simulink model "Lab2_Task_4"  (R2023b)
settings: Solver=FixedStepDiscrete  StartTime=0.0  StopTime=Inf  FixedStep=0.02  RelTol=1e-3  EnableMultiTasking=on
model workspace (MAT data in the model file):
  SL_ROS_VariableLengthArrays_MaxSizes.CommonInfo.ArrayTruncateAction = 'EmitWarning'
  SL_ROS_VariableLengthArrays_MaxSizes.MsgTypeMap = containers.Map
  SL_ROS_VariableLengthArrays_MaxSizes.MsgTypeMap.serialization.keys = {'sensor_msgs/LaserScan'}
  SL_ROS_VariableLengthArrays_MaxSizes.MsgTypeMap.serialization.values{1}(1).PropertyName = 'Intensities'
  SL_ROS_VariableLengthArrays_MaxSizes.MsgTypeMap.serialization.values{1}(1).DataType = 'single'
  SL_ROS_VariableLengthArrays_MaxSizes.MsgTypeMap.serialization.values{1}(1).MaxLength = 360
  SL_ROS_VariableLengthArrays_MaxSizes.MsgTypeMap.serialization.values{1}(2).PropertyName = 'Ranges'
  SL_ROS_VariableLengthArrays_MaxSizes.MsgTypeMap.serialization.values{1}(2).DataType = 'single'
  SL_ROS_VariableLengthArrays_MaxSizes.MsgTypeMap.serialization.values{1}(2).MaxLength = 360
  SL_ROS_VariableLengthArrays_MaxSizes.MsgTypeMap.serialization.uniformity = 0
  SL_ROS_VariableLengthArrays_MaxSizes.MsgTypeMap.serialization.keyType = 'char'
  SL_ROS_VariableLengthArrays_MaxSizes.MsgTypeMap.serialization.valueType = 'any'
undefined symbols (not defined in the file or in its folder): angdiff, Angular, DiscIntNeverNeededParam, Linear
libraries: robotlib x3, simulink_extras x2, robotcorelib x1
settings Model: Creator=The MathWorks, Inc.  LastModifiedBy=hampu
settings SolverCC: AlgebraicLoopSolver=TrustRegion
settings DataIOCC: LimitDataPoints=on  SaveFormat=Array  ReturnWorkspaceOutputs=off
settings OptimizationCC: ZeroExternalMemoryAtStartup=off  ZeroInternalMemoryAtStartup=off  LifeSpan=Inf  MaxStackSize=64
settings DebuggingCC: SolverPrmCheckMsg=warning  UnconnectedInputMsg=warning  UnconnectedOutputMsg=warning  UnconnectedLineMsg=warning  AllowSymbolicDim=off  SFUnexpectedBacktrackingDiag=warning  SFNoUnconditionalDefaultTransitionDiag=warning  SFExecutionAtInitializationDiag=none  ArithmeticOperatorsInVariantConditions=warning
settings HardwareCC: ProdBitPerPointer=32  ProdBitPerSizeT=32  ProdBitPerPtrDiffT=32  ProdLargestAtomicFloat=None  ProdIntDivRoundTo=Undefined  ProdEndianess=Unspecified  ProdWordSize=32  ProdHWDeviceType=Generic->Unspecified (assume 32-bit Generic)  TargetHWDeviceType=Generic->Unspecified (assume 32-bit Generic)  UseEmbeddedCoderFeatures=off
settings ModelReferenceCC: EnableRefExpFcnMdlSchedulingChecks=on  PropagateSignalLabelsOutOfModel=off
settings SFSimCC: SimUseLocalCustomCode=off  CustomCodeUndefinedFunction=UseInterfaceOnly  SimTargetLang=C++
settings RTWCC: Description=Embedded Coder  SystemTargetFile=ert.tlc  HardwareBoard=Robot Operating System (ROS)  TemplateMakefile=ert_default_tmf  RTWUseLocalCustomCode=off  Toolchain=Catkin  TargetLang=C++
settings CodeAppCC: StateflowObjectComments=on
settings ERTTargetCC: MultiwordLength=2048  ERTCustomFileBanners=off  CodeInterfacePackaging=C++ class  SupportContinuousTime=on  SupportNonInlinedSFcns=on  RemoveResetFunc=off  SupportVariableSizeSignals=on  ModelStepFunctionPrototypeControlCompliant=off  RootIOFormat=Structure reference  ConvertIfToSwitch=off  SuppressUnreachableDefaultCases=off
settings ConfigComp: CovMetricSettings=dw  CovSaveCumulativeToWorkspaceVar=on  CovSaveSingleToWorkspaceVar=on  CovExternalEMLEnable=off  CovSFcnEnable=off

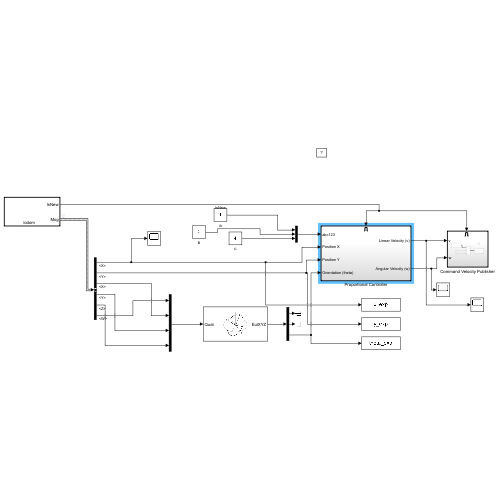
[thumbnail: Simulink's stored preview of the top-level diagram]
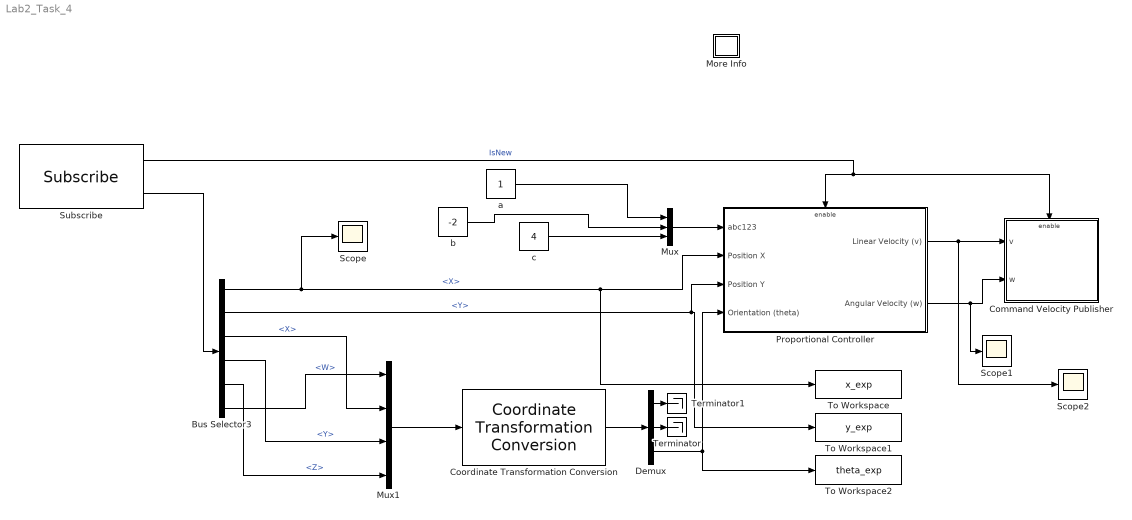
== system Lab2_Task_4 ==
  Bus Selector3 : BusSelector  OutputSignals=Pose.Pose.Position.X,Pose.Pose.Position.Y,Pose.Pose.Orientation.X,Pose.Pose.Orientation.Y,Pose.Pose.Orientation.Z,Pose.Pose.Orientation.W
  Command Velocity Publisher : Subsystem
  Coordinate Transformation Conversion : robotcorelib/Coordinate Transformation Conversion  InputRepresentation=Quaternion  InputEulerSequence=ZYX  ShowTrVecInputPort=on  OutputRepresentation=Euler Angles  OutputEulerSequence=XYZ  ShowTrVecOutputPort=on  SimulateUsing=Interpreted execution
      settings: LibrarySourceBlock=roslib/Utilities/Coordinate Transformation Conversion
  Demux : Demux  Outputs=3
  More Info : Subsystem
      settings: OpenFcn=showdemo(bdroot(gcb))
      mask Display: disp('?')
  Mux : Mux  Inputs=3
  Mux1 : Mux
  Proportional Controller : Subsystem
  Scope : Scope
  Scope1 : Scope
  Scope2 : Scope
  Subscribe : robotlib/Subscribe  topicSource=Select from ROS network  topic=/odom  messageType=nav_msgs/Odometry  SampleTime=-1  legacyBusStruct=off  messageQueueLength=51
  Terminator : Terminator
  Terminator1 : Terminator
  To Workspace : ToWorkspace  VariableName=x_exp  SaveFormat=Timeseries  SampleTime=-1
  To Workspace1 : ToWorkspace  VariableName=y_exp  SaveFormat=Timeseries  SampleTime=-1
  To Workspace2 : ToWorkspace  VariableName=theta_exp  SaveFormat=Timeseries  SampleTime=-1
  a : Constant
  b : Constant  Value=-2
  c : Constant  Value=4
  wires:
  Bus Selector3/5 -> Mux1/4  "<Z>"
  Bus Selector3/1 -> Scope/1, To Workspace/1, Proportional Controller/2(Position X)  "<X>"
  Mux1/1 -> Coordinate Transformation Conversion/1
  Proportional Controller/2(Angular Velocity (w)) -> Scope1/1, Command Velocity Publisher/2(w)
  Bus Selector3/4 -> Mux1/3  "<Y>"
  c/1 -> Mux/3
  Bus Selector3/2 -> To Workspace1/1, Proportional Controller/3(Position Y)  "<Y>"
  Coordinate Transformation Conversion/1 -> Demux/1
  Mux/1 -> Proportional Controller/1(abc123)
  Subscribe/1 -> Command Velocity Publisher/Enable, Proportional Controller/Enable  "IsNew"
  b/1 -> Mux/2
  Demux/2 -> Terminator/1
  Demux/3 -> Proportional Controller/4(Orientation (theta)), To Workspace2/1
  Bus Selector3/6 -> Mux1/1  "<W>"
  Proportional Controller/1(Linear Velocity (v)) -> Scope2/1, Command Velocity Publisher/1(v)
  Demux/1 -> Terminator1/1
  Subscribe/2 -> Bus Selector3/1
  a/1 -> Mux/1
  Bus Selector3/3 -> Mux1/2  "<X>"

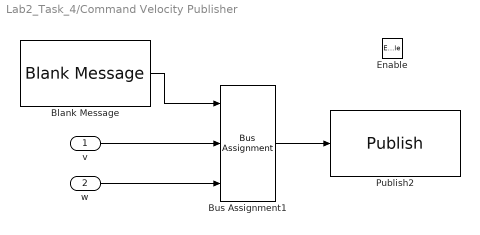
== system Lab2_Task_4/Command Velocity Publisher ==
  v : Inport
  w : Inport  Port=2
  Enable : EnablePort
  Blank Message : robotlib/Blank Message  messageClass=Message  entityType=geometry_msgs/Twist  messageType=geometry_msgs/Twist  SampleTime=inf  legacyBusStruct=off
  Bus Assignment1 : BusAssignment  DialogController=Simulink.DDGSource_BusAssignment  AssignedSignals=Linear.X,Angular.Z
  Publish2 : robotlib/Publish  topicSource=Select from ROS network  topic=/cmd_vel  messageType=geometry_msgs/Twist  legacyBusStruct=off  messageQueueLength=105
  wires:
  Bus Assignment1/1 -> Publish2/1
  Blank Message/1 -> Bus Assignment1/1
  v/1 -> Bus Assignment1/2
  w/1 -> Bus Assignment1/3

== system Lab2_Task_4/More Info ==

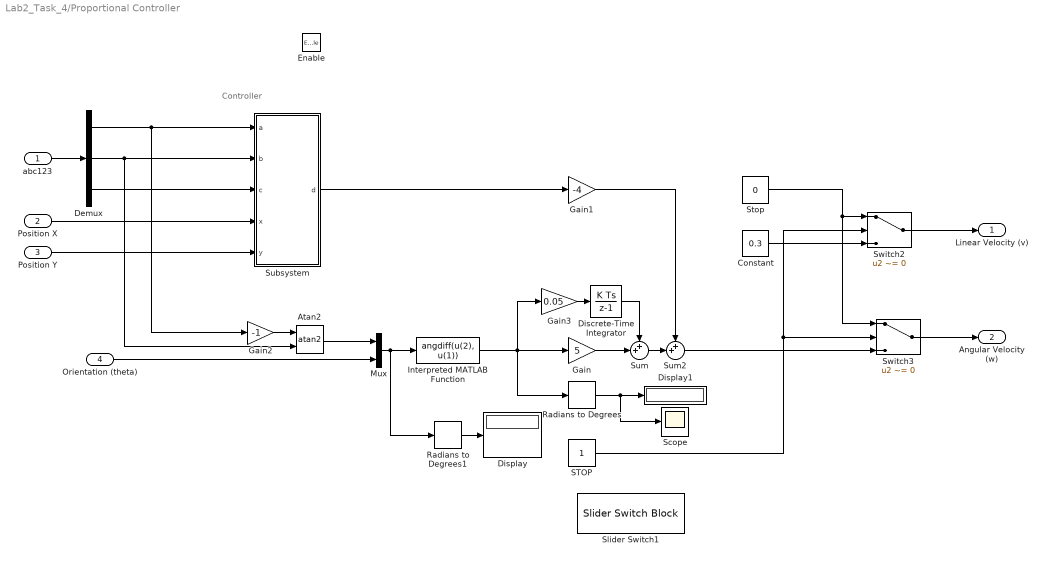
== system Lab2_Task_4/Proportional Controller ==
  note: Controller
  abc123 : Inport
  Position X : Inport  Port=2
  Position Y : Inport  Port=3
  Orientation (theta) : Inport  Port=4
  Enable : EnablePort
  Atan2 : Trigonometry  Operator=atan2
  Constant : Constant  Value=0.3
  Demux : Demux  Outputs=3
  Discrete-Time Integrator : DiscreteIntegrator  SampleTime=-1  ICPrevOutput=DiscIntNeverNeededParam  ICPrevScaledInput=DiscIntNeverNeededParam
  Display : Display
  Display1 : Display
  Gain : Gain  Gain=5
  Gain1 : Gain  Gain=-4
  Gain2 : Gain  Gain=-1
  Gain3 : Gain  Gain=0.05
  Interpreted MATLAB Function : MATLABFcn  MATLABFcn=angdiff(u(2), u(1))
  Mux : Mux  Inputs=2
  Radians to Degrees : simulink_extras/Transformations/Radians to Degrees
  Radians to Degrees1 : simulink_extras/Transformations/Radians to Degrees
  "STOP " : Constant
  Scope : Scope
  Slider Switch1 : SliderSwitchBlock
      settings: Values={{'on', 'off'}, [0 1]}
  Stop : Constant  Value=0
  Subsystem : Subsystem
  Sum : Sum  Inputs=++|
  Sum2 : Sum  Inputs=++|
  Switch2 : Switch  Criteria=u2 ~= 0  SaturateOnIntegerOverflow=off  InputSameDT=off
  Switch3 : Switch  Criteria=u2 ~= 0  SaturateOnIntegerOverflow=off  InputSameDT=off
  Linear Velocity (v) : Outport  VectorParamsAs1DForOutWhenUnconnected=off
  Angular Velocity (w) : Outport  Port=2  VectorParamsAs1DForOutWhenUnconnected=off
  wires:
  Stop/1 -> Switch3/1, Switch2/1
  "STOP "/1 -> Switch2/2, Switch3/2
  Switch2/1 -> Linear Velocity (v)/1
  Switch3/1 -> Angular Velocity (w)/1
  Gain/1 -> Sum/2
  Gain1/1 -> Sum2/1
  Sum2/1 -> Switch3/3
  Constant/1 -> Switch2/3
  Radians to Degrees/1 -> Scope/1, Display1/1
  Demux/2 -> Atan2/2, Subsystem/2(b)
  Demux/1 -> Gain2/1, Subsystem/1(a)
  abc123/1 -> Demux/1
  Gain2/1 -> Atan2/1
  Mux/1 -> Interpreted MATLAB Function/1, Radians to Degrees1/1
  Orientation (theta)/1 -> Mux/2
  Radians to Degrees1/1 -> Display/1
  Demux/3 -> Subsystem/3(c)
  Position X/1 -> Subsystem/4(x)
  Position Y/1 -> Subsystem/5(y)
  Subsystem/1(d) -> Gain1/1
  Atan2/1 -> Mux/1
  Interpreted MATLAB Function/1 -> Gain3/1, Radians to Degrees/1, Gain/1
  Discrete-Time Integrator/1 -> Sum/1
  Sum/1 -> Sum2/2
  Gain3/1 -> Discrete-Time Integrator/1

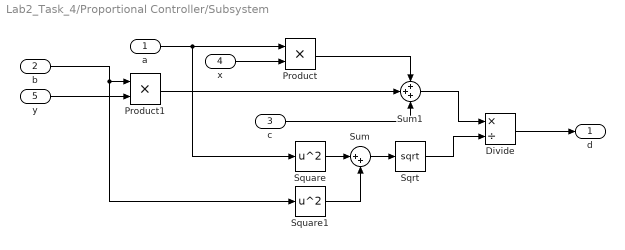
== system Lab2_Task_4/Proportional Controller/Subsystem ==
  a : Inport
  b : Inport  Port=2
  c : Inport  Port=3
  x : Inport  Port=4
  y : Inport  Port=5
  Divide : Product  Inputs=*/
  Product : Product
  Product1 : Product
  Sqrt : Sqrt
  Square : Math  Operator=square
  Square1 : Math  Operator=square
  Sum : Sum  Inputs=|++
  Sum1 : Sum  Inputs=+++
  d : Outport
  wires:
  Square1/1 -> Sum/2
  a/1 -> Square/1, Product/1
  b/1 -> Square1/1, Product1/1
  Product1/1 -> Sum1/2
  Sum/1 -> Sqrt/1
  Product/1 -> Sum1/1
  Square/1 -> Sum/1
  c/1 -> Sum1/3
  Sum1/1 -> Divide/1
  Divide/1 -> d/1
  Sqrt/1 -> Divide/2
  y/1 -> Product1/2
  x/1 -> Product/2
